simulink model "Test14Dof"  (R2024a)
settings: Solver=ode4  StartTime=0.0  StopTime=10.0  FixedStep=0.001  RelTol=1e-3
values from neighbouring files (symbols this model uses):
  EnvGrvty = 9.81    [Par.m]
  PlntBattChrgMax = 4.493    [Par.m]
  PlntBattNumCellSer = 96    [Par.m]
  PlntBattOpenCirctVolt = [3.17242 3.17242 3.17242 3.17242 3.17242 3.17242 3.17242;3.18272 3.18272 3.18272 3.18272 3.18272 3.18272 3.18272;3.19302 3.19302 3.19302 3.19302 3.19302 3.19302 3.19302;3.20331 3.20331 3.20331 3.20331 3.20331 3.20331 3.20331;3.21361 3.21361 3.21361 3.21361 3.21361 3.21361 3.21361;3.22391 3.22391 3.22391 3.22391 3.22391 3.22391 3.22391;3.23421 3.23421 3.23421 3.23421 3.23421 3.23421 3.23421;3.24451 ...(+5187 chars)    [Par.m]
  PlntBattSocInit = 0.6    [Par.m]
  PlntBattTempBpt = [-40 -30 -20 0 23 45 60]    [Par.m]
  PlntBattTempInitDegC = 25    [Par.m]
  PlntBattVoltSocBpt = [0 0.01 0.02 0.03 0.04 0.05 0.06 0.07 0.08 0.09 0.1 0.11 0.12 0.13 0.14 0.15 0.16 0.17 0.18 0.19 0.2 0.21 0.22 0.23 0.24 0.25 0.26 0.27 0.28 0.29 0.3 0.31 0.32 0.33 0.34 0.35 0.36 0.37 0.38 0.39 0.4 0.41 0.42 0.43 0.44 0.45 0.46 0.47 0.48 0.49 0.5 0.51 0.52 0.53 0.54 0.55 0.56 0.57 0.58 0.59 0.6 0.61 0.62 0.63 0.64 0.65 0.66 0.67 0.68 0.69 0.7 0.71 0.72 0.73 0.74 0.75 0.76 0.77 0.78 0.79 0.8 0.81  ...(+91 chars)    [Par.m]
  PlntDCDCVoltInit = 650    [Par.m]
  PlntDriveshftDamp = 100    [Par.m]
  PlntDriveshftStiff = 500    [Par.m]
  PlntEM1RotDamp = 0.001    [Par.m]
  PlntEM1RotInertia = 0.01    [Par.m]
  PlntEM2RotDamp = 0.001    [Par.m]
  PlntEM2RotInertia = 0.01    [Par.m]
  PlntEM3RotDamp = 0.001    [Par.m]
  PlntEM3RotInertia = 0.01    [Par.m]
  PlntEM4RotDamp = 0.001    [Par.m]
  PlntEM4RotInertia = 0.01    [Par.m]
  PlntEMWhlGearRatioFL = 11.04    [Par.m]
  PlntEMWhlGearRatioFR = 11.04    [Par.m]
  PlntEMWhlGearRatioRL = 11.04    [Par.m]
  PlntEMWhlGearRatioRR = 11.04    [Par.m]
  PlntSteerGearRatio = 52.025    [Par.m]
  PlntVehCGHgtAxl = 0.375    [Par.m]
  PlntVehDstCGFrntAxl = 1.61    [Par.m]
  PlntVehDstCGRearAxl = 1.39    [Par.m]
  PlntVehFrntUnsprgMass = 100    [Par.m]
  PlntVehInitLatPos = 0    [Par.m]
  PlntVehInitLatVel = 0    [Par.m]
  PlntVehInitLongPos = 0    [Par.m]
  PlntVehInitLongVel = 0    [Par.m]
  PlntVehInitPitchAng = 0    [Par.m]
  PlntVehInitPitchRate = 0    [Par.m]
  PlntVehInitRollAng = 0    [Par.m]
  PlntVehInitRollRate = 0    [Par.m]
  PlntVehInitVertPos = 0    [Par.m]
  PlntVehInitVertVel = 0    [Par.m]
  PlntVehInitYawAng = 0    [Par.m]
  PlntVehInitYawRate = 0    [Par.m]
  PlntVehMass = 2497    [Par.m]
  PlntVehPitchMomentInertia = 1922.7    [Par.m]
  PlntVehRearUnsprgMass = 100    [Par.m]
  PlntVehRollMomentInertia = 432.33333333333331    (= 432.333333333)    [Par.m]
  PlntVehTrckWdth = [1.685,1.685]    [Par.m]
  PlntVehYawMomentInertia = 2066    [Par.m]
  PlntWhlNumFrnt = 2    [Par.m]
  PlntWhlNumRear = 2    [Par.m]
  PlntWhlPrsFrnt = 220000    [Par.m]
  PlntWhlPrsRear = 220000    [Par.m]
undefined symbols (not defined in the file or in its folder): BdyFrm, InertFrm, PlntTrnsfrCaseAxlSpdLock, PlntTrnsfrCaseTrqSplitRatio
libraries: autolibsharedcoupling x12, autolibsharedcommon x12, autolibutils x10, autolibmappedmotor x4, autolibcoupling x4, matrix_library x4, vehdynlibsuspension x2, vehdynlibtire x2, vehdynlibtirecommon x2, vehdynlibsteering x2, shared6dof x2, autolibdatasheetbattery x1
(part 1 of 7)
settings Model: DataDictionary=VirtualVehicleTemplate.sldd  Creator=admin  LastModifiedBy=admin

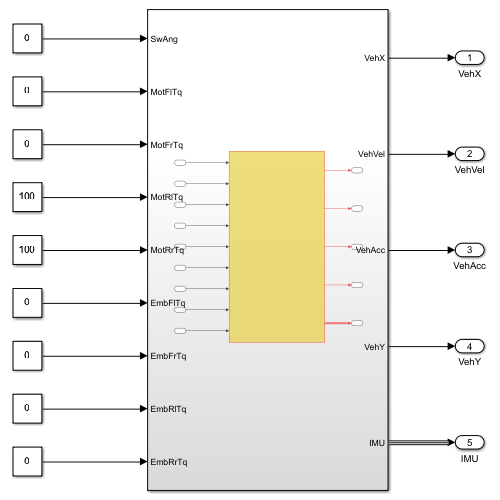
[thumbnail: Simulink's stored preview of the top-level diagram]
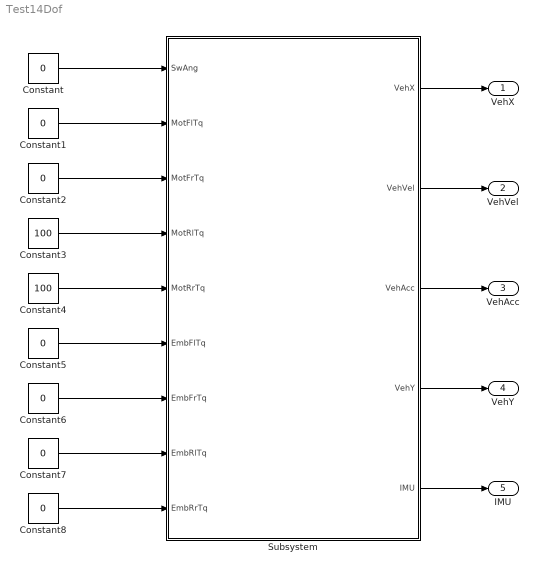
== system Test14Dof ==
  Constant{,1..2,5..8} (7 alike) : Constant  Value=0
  Constant3 : Constant  Value=100
  Constant4 : Constant  Value=100
  Subsystem : Subsystem
  VehX : Outport
  VehVel : Outport  Port=2
  VehAcc : Outport  Port=3
  VehY : Outport  Port=4
  IMU : Outport  Port=5
  wires:
  Subsystem/1(VehX) -> VehX/1
  Constant6/1 -> Subsystem/7(EmbFrTq)
  Constant5/1 -> Subsystem/6(EmbFlTq)
  Constant4/1 -> Subsystem/5(MotRrTq)
  Subsystem/3(VehAcc) -> VehAcc/1
  Constant2/1 -> Subsystem/3(MotFrTq)
  Constant/1 -> Subsystem/1(SwAng)
  Constant3/1 -> Subsystem/4(MotRlTq)
  Constant1/1 -> Subsystem/2(MotFlTq)
  Constant7/1 -> Subsystem/8(EmbRlTq)
  Subsystem/5(IMU) -> IMU/1
  Constant8/1 -> Subsystem/9(EmbRrTq)
  Subsystem/2(VehVel) -> VehVel/1
  Subsystem/4(VehY) -> VehY/1

== system Test14Dof/Subsystem ==
  SwAng : Inport
  MotFlTq : Inport  Port=2
  MotFrTq : Inport  Port=3
  MotRlTq : Inport  Port=4
  MotRrTq : Inport  Port=5
  EmbFlTq : Inport  Port=6
  EmbFrTq : Inport  Port=7
  EmbRlTq : Inport  Port=8
  EmbRrTq : Inport  Port=9
  Vehicle 14 DoF model : Subsystem
  VehX : Outport
  VehVel : Outport  Port=2
  VehAcc : Outport  Port=3
  VehY : Outport  Port=4
  IMU : Outport  Port=5
  wires:
  MotRrTq/1 -> Vehicle 14 DoF model/5(MotRrTq)
  MotFrTq/1 -> Vehicle 14 DoF model/3(MotFrTq)
  SwAng/1 -> Vehicle 14 DoF model/1(SwAng)
  MotRlTq/1 -> Vehicle 14 DoF model/4(MotRlTq)
  MotFlTq/1 -> Vehicle 14 DoF model/2(MotFlTq)
  EmbRlTq/1 -> Vehicle 14 DoF model/8(EmbRlTq)
  Vehicle 14 DoF model/3(VehAcc) -> VehAcc/1
  EmbFlTq/1 -> Vehicle 14 DoF model/6(EmbFlTq)
  Vehicle 14 DoF model/5(IMU) -> IMU/1
  EmbFrTq/1 -> Vehicle 14 DoF model/7(EmbFrTq)
  EmbRrTq/1 -> Vehicle 14 DoF model/9(EmbRrTq)
  Vehicle 14 DoF model/1(VehX) -> VehX/1
  Vehicle 14 DoF model/2(VehVel) -> VehVel/1
  Vehicle 14 DoF model/4(VehY) -> VehY/1

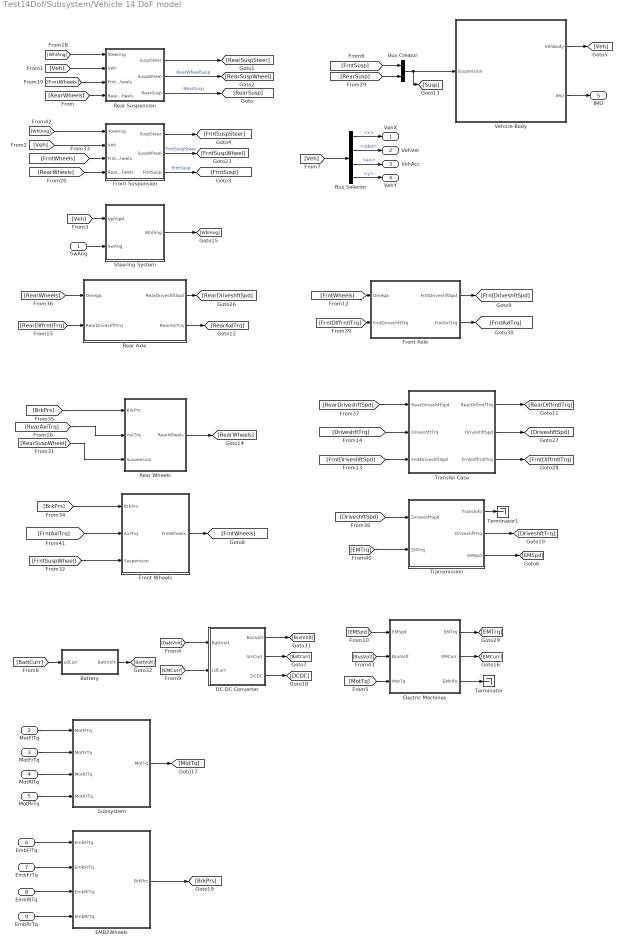
== system Test14Dof/Subsystem/Vehicle 14 DoF model ==
  SwAng : Inport
  MotFlTq : Inport  Port=2
  MotFrTq : Inport  Port=3
  MotRlTq : Inport  Port=4
  MotRrTq : Inport  Port=5
  EmbFlTq : Inport  Port=6
  EmbFrTq : Inport  Port=7
  EmbRlTq : Inport  Port=8
  EmbRrTq : Inport  Port=9
  Battery : Subsystem
  Bus Creator : BusCreator  Inputs=2
  Bus Selector : BusSelector  OutputSignals=BdyFrm.Cg.Disp.x,BdyFrm.Cg.Vel.xdot,BdyFrm.Cg.Acc.ax,BdyFrm.Cg.Disp.y
  DC-DC Converter : Subsystem
  EMB2Wheels : Subsystem
  Electric Machines : Subsystem
  Front Axle : Subsystem
  Front Suspension : Subsystem
  Front Wheels : Subsystem
  Rear Axle : Subsystem
  Rear Suspension : Subsystem
  Rear Wheels : Subsystem
  Steering System : Subsystem
  Subsystem : Subsystem
  Terminator : Terminator
  Terminator1 : Terminator
  Transfer Case : Subsystem
  Transmission : Subsystem
  Vehicle Body : Subsystem
  VehX : Outport
  VehVel : Outport  Port=2
  VehAcc : Outport  Port=3
  VehY : Outport  Port=4
  IMU : Outport  Port=5
  wires:
  EmbRrTq/1 -> EMB2Wheels/4(EmbRrTq)
  [FrntSuspWheel] -> Front Wheels/3(Suspension)
  Subsystem/1(MotTq) -> [MotTq]
  [FrntDiffrntlTrq] -> Front Axle/2(FrntDriveshftTrq)
  Transmission/3(EMSpd) -> [EMSpd]
  [FrntWheels] -> Rear Suspension/3(FrntWheels)
  MotRlTq/1 -> Subsystem/3(MotRlTq)
  EmbFlTq/1 -> EMB2Wheels/1(EmbFlTq)
  SwAng/1 -> Steering System/2(SwAng)
  [BrkPrs] -> Front Wheels/1(BrkPrs)
  [RearSusp] -> Bus Creator/2
  MotFrTq/1 -> Subsystem/2(MotFrTq)
  Electric Machines/1(EMTrq) -> [EMTrq]
  [RearDiffrntlTrq] -> Rear Axle/2(RearDriveshftTrq)
  Front Wheels/1(FrntWheels) -> [FrntWheels]
  Front Suspension/3(FrntSusp) -> [FrntSusp]  "FrntSusp"
  DC-DC Converter/2(SrcCurr) -> [BattCurr]
  [EMTrq] -> Transmission/2(EMTrq)
  [FrntWheels] -> Front Axle/1(Omega)
  [BusVolt] -> Electric Machines/2(BusVolt)
  [WhlAng] -> Rear Suspension/1(Steering)
  Front Suspension/2(SuspWheel) -> [FrntSuspWheel]  "FrntSuspSteer"
  Front Axle/1(FrntDriveshftSpd) -> [FrntDriveshftSpd]
  [BattCurr] -> Battery/1(LdCurr)
  Front Suspension/1(SuspSteer) -> [FrntSuspSteer]
  Vehicle Body/1(VehBody) -> [Veh]
  [MotTq] -> Electric Machines/3(MotTq)
  [RearWheels] -> Rear Axle/1(Omega)
  [FrntDriveshftSpd] -> Transfer Case/3(FrntDriveshftSpd)
  Battery/1(BattVolt) -> [BattVolt]
  Rear Axle/2(RearAxlTrq) -> [RearAxlTrq]
  [EMSpd] -> Electric Machines/1(EMSpd)
  [DriveshftSpd] -> Transmission/1(DriveshftSpd)
  [Veh] -> Steering System/1(VehSpd)
  [EMCurr] -> DC-DC Converter/2(LdCurr)
  Rear Wheels/1(RearWheels) -> [RearWheels]
  [RearWheels] -> Rear Suspension/4(RearWheels)
  Bus Creator/1 -> Vehicle Body/1(Suspension), [Susp]
  Transmission/2(DriveshftTrq) -> [DriveshftTrq]
  EmbFrTq/1 -> EMB2Wheels/2(EmbFrTq)
  Rear Suspension/2(SuspWheel) -> [RearSuspWheel]  "RearWheelSusp"
  [BattVolt] -> DC-DC Converter/1(BattVolt)
  [Veh] -> Rear Suspension/2(Veh)
  [DriveshftTrq] -> Transfer Case/2(DriveshftTrq)
  [BrkPrs] -> Rear Wheels/1(BrkPrs)
  MotRrTq/1 -> Subsystem/4(MotRrTq)
  Steering System/1(WhlAng) -> [WhlAng]
  Rear Suspension/1(SuspSteer) -> [RearSuspSteer]
  Transfer Case/2(DriveshftSpd) -> [DriveshftSpd]
  EMB2Wheels/1(BrkPrs) -> [BrkPrs]
  MotFlTq/1 -> Subsystem/1(MotFlTq)
  [RearDriveshftSpd] -> Transfer Case/1(RearDriveshftSpd)
  Transfer Case/3(FrntDiffrntlTrq) -> [FrntDiffrntlTrq]
  Electric Machines/2(EMCurr) -> [EMCurr]
  Front Axle/2(FrntAxlTrq) -> [FrntAxlTrq]
  [FrntSusp] -> Bus Creator/1
  EmbRlTq/1 -> EMB2Wheels/3(EmbRlTq)
  Rear Suspension/3(RearSusp) -> [RearSusp]  "RearSusp"
  DC-DC Converter/1(BusVolt) -> [BusVolt]
  [RearAxlTrq] -> Rear Wheels/2(AxlTrq)
  DC-DC Converter/3(DCDC) -> [DCDC]
  [RearSuspWheel] -> Rear Wheels/3(Suspension)
  Rear Axle/1(RearDriveshftSpd) -> [RearDriveshftSpd]
  [FrntAxlTrq] -> Front Wheels/2(AxlTrq)
  Transfer Case/1(RearDiffrntlTrq) -> [RearDiffrntlTrq]
  Transmission/1(TransInfo) -> Terminator1/1
  Electric Machines/3(EMInfo) -> Terminator/1
  [Veh] -> Front Suspension/2(Veh)
  [RearWheels] -> Front Suspension/4(RearWheels)
  [FrntWheels] -> Front Suspension/3(FrntWheels)
  [WhlAng] -> Front Suspension/1(Steering)
  [Veh] -> Bus Selector/1
  Bus Selector/1 -> VehX/1  "<x>"
  Bus Selector/2 -> VehVel/1  "<xdot>"
  Bus Selector/3 -> VehAcc/1  "<ax>"
  Bus Selector/4 -> VehY/1  "<y>"
  Vehicle Body/2(IMU) -> IMU/1

== system Test14Dof/Subsystem/Vehicle 14 DoF model/Battery ==
  LdCurr : Inport
  Constant : Constant  Value=27
  Fcn : Fcn  Expr=u+273
  Lithium Ion Battery Pack : autolibdatasheetbattery/Datasheet Battery  CapacityCtrl=Parameter  OutputVlt=Filtered  BattChargeMax=PlntBattChrgMax  Em=interp2(PlntBattTempBpt,PlntBattVoltSocBpt',PlntBattOpenCirctVolt,PlntBattTempInitDegC,PlntBattVoltSocBpt')'  CapLUTBp=PlntBattVoltSocBpt  RInt=PlntBattIntrnRes'  BattTempBp=PlntBattTempBpt+273.15  CapSOCBp=PlntBattSocBpt  Ns=PlntBattNumCellSer  Np=PlntBattNumCellPar  BattCapInit=PlntBattSocInit*PlntBattChrgMax  Tc=PlntBattTimeCnst  Vinit=interp2(PlntBattTempBpt,PlntBattVoltSocBpt,PlntBattOpenCirctVolt*PlntBattNumCellSer,PlntBattTempInitDegC,PlntBattSocInit)  RefBlkName='autolibdatasheetbattery/Datasheet Battery'
  BattVolt : Outport  VectorParamsAs1DForOutWhenUnconnected=off
  wires:
  Lithium Ion Battery Pack/2 -> BattVolt/1
  Constant/1 -> Fcn/1
  Fcn/1 -> Lithium Ion Battery Pack/2
  LdCurr/1 -> Lithium Ion Battery Pack/1  "TotalCurr"

== system Test14Dof/Subsystem/Vehicle 14 DoF model/DC-DC Converter ==
  BattVolt : Inport
  LdCurr : Inport  Port=2
  Bus Selector1 : BusSelector  OutputSignals=PwrLoss  OutputAsBus=on
  Constant3 : Constant  Value=PlntDCDCVoltInit  SampleTime=-1
  Cont LPF : autolibutils/Cont LPF  wc=1  AbsoluteTolerance=auto  aMode=6
  DC-DC Converter : autolibdcdc/Bidirectional DC-DC  Tc=PlntDCDCTimeCnst  Vinit=PlntDCDCVoltInit  Plimit=PlntDCDCPwrLmt  param_loss=Single efficiency measurement  eff=PlntDCDCEff  v_loss_bp=PlntDCDCLossV  i_loss_bp=PlntDCDCLossI  losses_table=PlntDCDCLossTbl  v_eff_bp=[200 400 600 800 1000]  i_eff_bp=[25 50 75 100]  efficiency_table=[96.2 98.1 98.7 99;98.1 99 99.4 99.5;98.7 99.4 99.6 99.7;99 99.5 99.7 99.8;99.2 99.6 99.7 99.8]  x_v_bp=[-1000 -800 -600 -400 -200 200 400 600 800 1000]  x_i_bp=[-100 -75 -50 -25 25 50 75 100]  x_losses_mat=[200.400801603196 225.67703109328 200.803212851408 201.612903225806 199.999999999997 200 225 200;160.320641282556 180.541624874624 201.005025125625 202.020202020203 200 200 180 160;180.541624874624 180.722891566267 181.086519114686 197.568389057748 194.999999999999 179.999999999997 180 180;201.005025125625 181.086519114686 202.020202020203 193.67991845056 190 200 179.999999999997 200;202.020202020203 197.568389057748 193.67991845056 197.505197505197 190 190 194.999999999999 200;200 194.999999999999 190 190 197.505197505197 193.67991845056 197.568389057748 202.020202020203;200 179.999999999997 200 190 193.67991845056 202.020202020203 181.086519114686 201.005025125625;180 180 179.999999999997 194.999999999999 197.568389057748 181.086519114686 180.722891566267 180.541624874624;160 180 200 200 202.020202020203 201.005025125625 180.541624874624 160.320641282556;200 225 200 199.999999999997 201.612903225806 200.803212851408 225.67703109328 200.400801603196]  RefBlkName='autolibdcdc/Bidirectional DC-DC'  CalLossMapData={'BaseCageProjectFileName','';'BaseMbcProjectFileName','';'TaskName','Calibrate Inverter Loss Map';'ChildTasks',{{'DataName','';'TaskName','Import Loss Data'},{'TaskName','Generate Response Models'},{'TaskName','Generate Calibration'},{'TaskName','Update Block Parameters'}}}
  BusVolt : Outport  VectorParamsAs1DForOutWhenUnconnected=off
  SrcCurr : Outport  Port=2  VectorParamsAs1DForOutWhenUnconnected=off
  Bus Element Out : Outport  Port=3  PortName=DCDC  Element=PwrELoss
  wires:
  Cont LPF/1 -> Bus Element Out/1
  Bus Selector1/1 -> Cont LPF/1
  LdCurr/1 -> DC-DC Converter/3
  BattVolt/1 -> DC-DC Converter/2
  DC-DC Converter/2 -> BusVolt/1
  DC-DC Converter/1 -> Bus Selector1/1
  Constant3/1 -> DC-DC Converter/1
  DC-DC Converter/3 -> SrcCurr/1

== system Test14Dof/Subsystem/Vehicle 14 DoF model/EMB2Wheels ==
  EmbFlTq : Inport
  EmbFrTq : Inport  Port=2
  EmbRlTq : Inport  Port=3
  EmbRrTq : Inport  Port=4
  Bus Creator : BusCreator  Inputs=4
  Gain{,1..3} (4 alike) : Gain
  Transfer Fcn{,1..3} (4 alike) : TransferFcn  Denominator=[0.01 1]
  BrkPrs : Outport
  wires:
  EmbRrTq/1 -> Gain1/1
  EmbFlTq/1 -> Gain/1
  EmbRlTq/1 -> Gain3/1
  EmbFrTq/1 -> Gain2/1
  Gain2/1 -> Transfer Fcn2/1
  Gain/1 -> Transfer Fcn/1
  Transfer Fcn3/1 -> Bus Creator/3
  Gain1/1 -> Transfer Fcn1/1
  Gain3/1 -> Transfer Fcn3/1
  Transfer Fcn/1 -> Bus Creator/1
  Transfer Fcn2/1 -> Bus Creator/2
  Transfer Fcn1/1 -> Bus Creator/4
  Bus Creator/1 -> BrkPrs/1

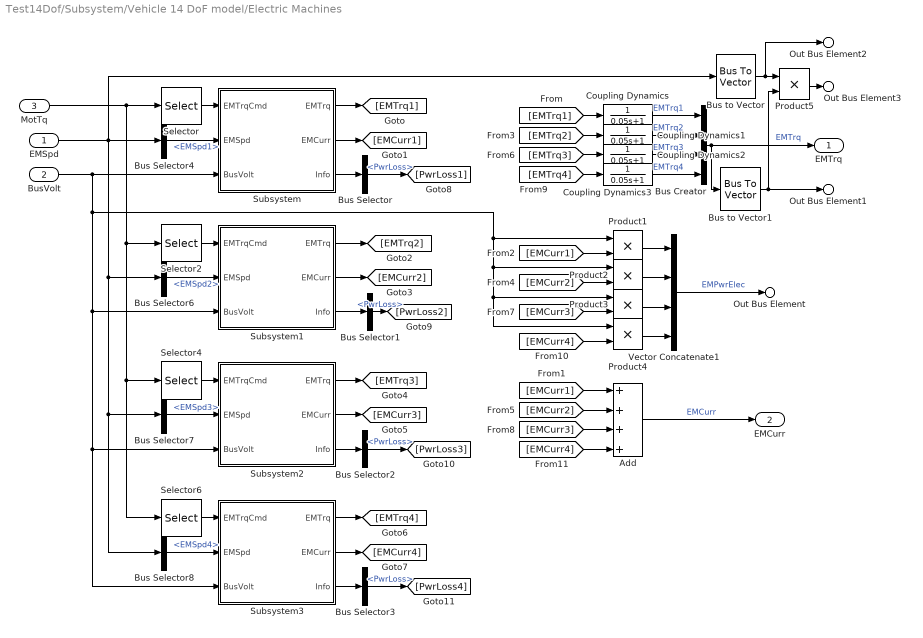
== system Test14Dof/Subsystem/Vehicle 14 DoF model/Electric Machines ==
  EMSpd : Inport
  BusVolt : Inport  Port=2
  MotTq : Inport  Port=3
  Add : Sum  Inputs=++++
  Bus Creator : BusCreator  Inputs=4
  Bus Selector{,1..3} (4 alike) : BusSelector  OutputSignals=PwrLoss
  Bus Selector4 : BusSelector  OutputSignals=EMSpd1
  Bus Selector6 : BusSelector  OutputSignals=EMSpd2
  Bus Selector7 : BusSelector  OutputSignals=EMSpd3
  Bus Selector8 : BusSelector  OutputSignals=EMSpd4
  Bus to Vector : BusToVector
  Bus to Vector1 : BusToVector
  Coupling Dynamics{,1..3} (4 alike) : TransferFcn  Denominator=[0.05 1]
  Product{1..5} (5 alike) : Product
  Selector : Selector  InputPortWidth=4  IndexOptions=Index vector (dialog)  Indices=[1]  OutputSizes=1
  Selector2 : Selector  InputPortWidth=4  IndexOptions=Index vector (dialog)  Indices=[2]  OutputSizes=1
  Selector4 : Selector  InputPortWidth=4  IndexOptions=Index vector (dialog)  Indices=[3]  OutputSizes=1
  Selector6 : Selector  InputPortWidth=4  IndexOptions=Index vector (dialog)  Indices=[4]  OutputSizes=1
  Subsystem : Subsystem
  Subsystem1 : Subsystem
  Subsystem2 : Subsystem
  Subsystem3 : Subsystem
  Vector Concatenate1 : Concatenate  NumInputs=4
  EMTrq : Outport
  EMCurr : Outport  Port=2
  Out Bus Element : Outport  Port=3  PortName=EMInfo  Element=EMPwrElec
  Out Bus Element1 : Outport  Port=3  PortName=EMInfo  Element=EMTrq
  Out Bus Element2 : Outport  Port=3  PortName=EMInfo  Element=EMSpd
  Out Bus Element3 : Outport  Port=3  PortName=EMInfo  Element=EMMechPwr
  wires:
  Bus Selector4/1 -> Subsystem/2(EMSpd)  "<EMSpd1>"
  [EMCurr2] -> Add/2
  Bus Selector1/1 -> [PwrLoss2]  "<PwrLoss>"
  [EMCurr3] -> Add/3
  [EMCurr2] -> Product2/2
  Product4/1 -> Vector Concatenate1/4
  Subsystem1/3(Info) -> Bus Selector1/1
  Bus Selector3/1 -> [PwrLoss4]  "<PwrLoss>"
  [EMCurr3] -> Product3/2
  Bus Selector6/1 -> Subsystem1/2(EMSpd)  "<EMSpd2>"
  Subsystem3/1(EMTrq) -> [EMTrq4]
  Subsystem2/3(Info) -> Bus Selector2/1
  Selector2/1 -> Subsystem1/1(EMTrqCmd)
  [EMTrq3] -> Coupling Dynamics2/1
  Selector4/1 -> Subsystem2/1(EMTrqCmd)
  Coupling Dynamics2/1 -> Bus Creator/3  "EMTrq3"
  Bus Selector/1 -> [PwrLoss1]  "<PwrLoss>"
  Subsystem3/3(Info) -> Bus Selector3/1
  Bus Selector2/1 -> [PwrLoss3]  "<PwrLoss>"
  Bus Selector7/1 -> Subsystem2/2(EMSpd)  "<EMSpd3>"
  Subsystem2/1(EMTrq) -> [EMTrq3]
  BusVolt/1 -> Subsystem/3(BusVolt), Subsystem1/3(BusVolt), Subsystem3/3(BusVolt), Subsystem2/3(BusVolt), Product1/1, Product4/1, Product3/1, Product2/1
  [EMCurr1] -> Product1/2
  Subsystem1/1(EMTrq) -> [EMTrq2]
  MotTq/1 -> Selector6/1, Selector4/1, Selector2/1, Selector/1
  Bus to Vector1/1 -> Product5/2, Out Bus Element1/1
  [EMCurr4] -> Add/4
  Product3/1 -> Vector Concatenate1/3
  [EMTrq4] -> Coupling Dynamics3/1
  Subsystem2/2(EMCurr) -> [EMCurr3]
  Subsystem/3(Info) -> Bus Selector/1
  Coupling Dynamics/1 -> Bus Creator/1  "EMTrq1"
  EMSpd/1 -> Bus Selector4/1, Bus Selector6/1, Bus Selector8/1, Bus Selector7/1, Bus to Vector/1
  Selector6/1 -> Subsystem3/1(EMTrqCmd)
  [EMCurr4] -> Product4/2
  Product5/1 -> Out Bus Element3/1
  Subsystem/1(EMTrq) -> [EMTrq1]
  Bus to Vector/1 -> Product5/1, Out Bus Element2/1
  Vector Concatenate1/1 -> Out Bus Element/1  "EMPwrElec"
  Product2/1 -> Vector Concatenate1/2
  Coupling Dynamics3/1 -> Bus Creator/4  "EMTrq4"
  Selector/1 -> Subsystem/1(EMTrqCmd)
  Subsystem/2(EMCurr) -> [EMCurr1]
  Product1/1 -> Vector Concatenate1/1
  Add/1 -> EMCurr/1  "EMCurr"
  [EMTrq1] -> Coupling Dynamics/1
  Bus Creator/1 -> Bus to Vector1/1, EMTrq/1  "EMTrq"
  [EMCurr1] -> Add/1
  Subsystem1/2(EMCurr) -> [EMCurr2]
  Bus Selector8/1 -> Subsystem3/2(EMSpd)  "<EMSpd4>"
  [EMTrq2] -> Coupling Dynamics1/1
  Subsystem3/2(EMCurr) -> [EMCurr4]
  Coupling Dynamics1/1 -> Bus Creator/2  "EMTrq2"

== system Test14Dof/Subsystem/Vehicle 14 DoF model/Front Axle ==
  Omega : Inport
  FrntDriveshftTrq : Inport  Port=2
  Bus Creator : BusCreator  Inputs=2
  Bus Selector : BusSelector  OutputSignals=Wheels.Omega
  Constant : Constant  Value=[0 0 0 0]
  Demux1 : Demux  Outputs=2
  Front Axle : Subsystem
  Front Axle Compliances : Subsystem
  Selector1 : Selector  InputPortWidth=4  IndexOptions=Index vector (dialog)  Indices=[3 4]  OutputSizes=1
  Subsystem : Subsystem
  FrntDriveshftSpd : Outport
  FrntAxlTrq : Outport  Port=2
  wires:
  Constant/1 -> Selector1/1
  Demux1/1 -> Front Axle/1(Prs1)
  Selector1/1 -> Demux1/1
  Demux1/2 -> Front Axle/2(Prs2)
  FrntDriveshftTrq/1 -> Front Axle/3(DriveshftTrq)
  Front Axle/2(DriveshftSpd) -> FrntDriveshftSpd/1
  Front Axle/3(Axl1Spd) -> Front Axle Compliances/1(RSpdL)
  Front Axle/4(Axl2Spd) -> Front Axle Compliances/2(RSpdR)
  Front Axle Compliances/2(RTrqR) -> Front Axle/5(Axl2Trq)
  Front Axle Compliances/1(RTrqL) -> Front Axle/4(Axl1Trq)
  Bus Selector/1 -> Subsystem/1(Omega)  "<Omega>"
  Omega/1 -> Bus Selector/1
  Subsystem/1(Omega_FL) -> Front Axle Compliances/3(OmegaL)
  Subsystem/2(Omega_FR) -> Front Axle Compliances/4(OmegaR)
  Front Axle Compliances/3(CTrqL) -> Bus Creator/1  "AxlTrqFL"
  Front Axle Compliances/4(CTrqR) -> Bus Creator/2  "AxlTrqFR"
  Bus Creator/1 -> FrntAxlTrq/1

== system Test14Dof/Subsystem/Vehicle 14 DoF model/Front Suspension ==
  Steering : Inport
  Veh : Inport  Port=2
  FrntWheels : Inport  Port=3
  RearWheels : Inport  Port=4
  Bus Creator : BusCreator  Inputs=2
  Bus Selector : BusSelector  OutputSignals=Wheels
  Bus Selector1 : BusSelector  OutputSignals=Wheels
  Kinematics and Compliance Independent Suspension : Subsystem
  Subsystem : Subsystem
  Susp2Wheel : Subsystem
  Wheel2Susp : Subsystem
  Wheel2SuspFrntOnly : Subsystem
  SuspSteer : Outport
  SuspWheel : Outport  Port=2
  FrntSusp : Outport  Port=3
  wires:
  Wheel2SuspFrntOnly/1(Wheels2Susp) -> SuspSteer/1
  FrntWheels/1 -> Bus Selector/1
  Kinematics and Compliance Independent Suspension/2(SuspensionFull) -> Susp2Wheel/1(Susp)
  Susp2Wheel/2(SuspFdbk) -> Wheel2Susp/3(SuspWheel)
  Bus Selector/1 -> Subsystem/1(Frnt), Susp2Wheel/3(Wheels), Wheel2SuspFrntOnly/2(Wheels)  "<Wheels>"
  Veh/1 -> Kinematics and Compliance Independent Suspension/2(Vehicle), Wheel2Susp/1(Veh), Wheel2SuspFrntOnly/1(Veh)
  Bus Creator/1 -> FrntSusp/1  "FrntSusp"
  RearWheels/1 -> Bus Selector1/1
  Subsystem/1(Wheels) -> Wheel2Susp/2(Wheels)
  Wheel2Susp/1(Wheels2Susp) -> Kinematics and Compliance Independent Suspension/3(Wheel), Susp2Wheel/2(WheelSusp)
  Steering/1 -> Kinematics and Compliance Independent Suspension/1(Steering)
  Bus Selector1/1 -> Subsystem/2(Rear)  "<Wheels>"
  Susp2Wheel/1(SuspWheel) -> SuspWheel/1, Bus Creator/2, Wheel2SuspFrntOnly/3(SuspWheel)  "FrntSuspWheel"
  Kinematics and Compliance Independent Suspension/1(Suspension) -> Bus Creator/1  "FrntSuspChassis"

== system Test14Dof/Subsystem/Vehicle 14 DoF model/Front Wheels ==
  BrkPrs : Inport
  AxlTrq : Inport  Port=2
  Suspension : Inport  Port=3
  Bus Creator1 : BusCreator  Inputs=2
  Bus Creator3 : BusCreator  Inputs=3
  Bus Selector : BusSelector  OutputSignals=Vx,Vy,WhlAng,YawRate,Fext
  Bus Creator : Subsystem
  Bus to Vector : BusToVector
  Constant : Constant  Value=[0.9 0.9 0.9 0.9]
  Constant1 : Constant  Value=[0 0 0 0]
  Constant2 : Constant  Value=repmat(eye(3),1,1,4)
  Front Friction : Subsystem
  Front Ground : Subsystem
  MF Tires Vector : Subsystem  VariantControl=MF Tires Vector
  Reshape : Reshape
  Selector : Selector  NumberOfDimensions=2  InputPortWidth=3  IndexOptions=Index vector (dialog),Select all  Indices=[1],1  OutputSizes=1,1
  Selector1 : Selector  NumberOfDimensions=3  IndexOptions=Index vector (dialog),Index vector (dialog),Index vector (dialog)  Indices=[1 2 3],[1 2 3],[1 2]  OutputSizes=1,1,1
  Selector4 : Selector  InputPortWidth=4  IndexOptions=Index vector (dialog)  Indices=[1 2]  OutputSizes=1
  Subsystem : Subsystem
  FrntWheels : Outport
  wires:
  Subsystem/2(ScaleFctrs) -> MF Tires Vector/9(ScaleFctrs)
  AxlTrq/1 -> Bus to Vector/1
  Bus to Vector/1 -> MF Tires Vector/2(AxlTrq)
  Selector1/1 -> Bus Creator3/3  "DCM"
  Bus Selector/2 -> MF Tires Vector/4(Vy)  "<Vy>"
  Front Friction/1(y) -> Subsystem/2(lamda_mu_y), Subsystem/1(lamda_mu_x), Bus Creator3/1  "mu"
  Reshape/1 -> MF Tires Vector/5(Camber)
  Subsystem/1(Prs) -> MF Tires Vector/8(Prs)
  Front Ground/1(y) -> MF Tires Vector/10(Gnd), Bus Creator3/2  "z"
  Selector4/1 -> MF Tires Vector/1(BrkPrs)
  Bus Selector/5 -> MF Tires Vector/7(Fext)  "<Fext>"
  Bus Selector/1 -> MF Tires Vector/3(Vx)  "<Vx>"
  Bus Selector/3 -> Selector/1  "<WhlAng>"
  Suspension/1 -> Bus Selector/1
  BrkPrs/1 -> Selector4/1
  Bus Selector/4 -> MF Tires Vector/6(YawRate)  "<YawRate>"
  Selector/1 -> Reshape/1
  Constant1/1 -> Front Ground/1(u)
  Constant/1 -> Front Friction/1(u)
  Constant2/1 -> Selector1/1
  Bus Creator1/1 -> FrntWheels/1
  Bus Creator/1(Wheels) -> Bus Creator1/1  "Wheels"
  MF Tires Vector/1(Wheels) -> Bus Creator/1(Info)
  Bus Creator3/1 -> Bus Creator1/2  "Gnd"

== system Test14Dof/Subsystem/Vehicle 14 DoF model/Rear Axle ==
  Omega : Inport
  RearDriveshftTrq : Inport  Port=2
  Bus Creator : BusCreator  Inputs=2
  Bus Selector : BusSelector  OutputSignals=Wheels.Omega
  Constant : Constant  Value=[0 0 0 0]
  Demux1 : Demux  Outputs=2
  Rear Axle : Subsystem
  Selector1 : Selector  InputPortWidth=4  IndexOptions=Index vector (dialog)  Indices=[3 4]  OutputSizes=1
  Subsystem : Subsystem
  Subsystem1 : Subsystem
  Terminator1 : Terminator
  RearDriveshftSpd : Outport
  RearAxlTrq : Outport  Port=2
  wires:
  Subsystem/1(RTrqL) -> Rear Axle/4(Axl1Trq)
  Bus Selector/1 -> Subsystem1/1(Omega)  "<Omega>"
  Omega/1 -> Bus Selector/1
  Demux1/2 -> Rear Axle/2(Prs2)
  Subsystem/2(RTrqR) -> Rear Axle/5(Axl2Trq)
  Selector1/1 -> Demux1/1
  RearDriveshftTrq/1 -> Rear Axle/3(DriveshftTrq)
  Demux1/1 -> Rear Axle/1(Prs1)
  Rear Axle/3(Axl1Spd) -> Subsystem/1(RSpdL)
  Rear Axle/4(Axl2Spd) -> Subsystem/2(RSpdR)
  Subsystem1/1(Omega_RL) -> Subsystem/3(OmegaL)
  Subsystem1/2(Omega_RR) -> Subsystem/4(OmegaR)
  Rear Axle/2(DriveshftSpd) -> RearDriveshftSpd/1
  Bus Creator/1 -> RearAxlTrq/1
  Subsystem/3(CTrqL) -> Bus Creator/1  "AxlTrqRL"
  Subsystem/4(CTrqR) -> Bus Creator/2  "AxlTrqRR"
  Constant/1 -> Selector1/1
  Rear Axle/1(Info) -> Terminator1/1

== system Test14Dof/Subsystem/Vehicle 14 DoF model/Rear Suspension ==
  note: Copyright 2022-2023 The MathWorks, Inc.
  Steering : Inport
  Veh : Inport  Port=2
  FrntWheels : Inport  Port=3
  RearWheels : Inport  Port=4
  Bus Creator : BusCreator  Inputs=2
  Bus Selector : BusSelector  OutputSignals=Wheels
  Bus Selector1 : BusSelector  OutputSignals=Wheels
  Kinematics and Compliance Independent Suspension : Subsystem
  Subsystem : Subsystem
  Susp2Wheel : Subsystem
  Wheel2Susp : Subsystem
  Wheel2SuspRearOnly : Subsystem
  SuspSteer : Outport
  SuspWheel : Outport  Port=2
  RearSusp : Outport  Port=3
  wires:
  Bus Selector1/1 -> Subsystem/2(Rear), Susp2Wheel/3(Wheels), Wheel2SuspRearOnly/2(Wheels)  "<Wheels>"
  Subsystem/1(Wheels) -> Wheel2Susp/2(Wheels)
  Kinematics and Compliance Independent Suspension/2(SuspensionFull) -> Susp2Wheel/1(Susp)
  RearWheels/1 -> Bus Selector1/1
  Susp2Wheel/2(SuspFdbk) -> Wheel2Susp/3(SuspWheel)
  Bus Creator/1 -> RearSusp/1  "RearSusp"
  Steering/1 -> Kinematics and Compliance Independent Suspension/1(Steering)
  Susp2Wheel/1(SuspWheel) -> Wheel2SuspRearOnly/3(SuspWheel), SuspWheel/1, Bus Creator/2  "RearSuspWheel"
  Wheel2SuspRearOnly/1(Wheels2Susp) -> SuspSteer/1
  Wheel2Susp/1(Wheels2Susp) -> Kinematics and Compliance Independent Suspension/3(Wheel), Susp2Wheel/2(WheelSusp)
  Bus Selector/1 -> Subsystem/1(Frnt)  "<Wheels>"
  FrntWheels/1 -> Bus Selector/1
  Kinematics and Compliance Independent Suspension/1(Suspension) -> Bus Creator/1  "RearSuspChassis"
  Veh/1 -> Kinematics and Compliance Independent Suspension/2(Vehicle), Wheel2Susp/1(Veh), Wheel2SuspRearOnly/1(Veh)

== system Test14Dof/Subsystem/Vehicle 14 DoF model/Rear Wheels ==
  BrkPrs : Inport
  AxlTrq : Inport  Port=2
  Suspension : Inport  Port=3
  Bus Creator1 : BusCreator  Inputs=2
  Bus Creator3 : BusCreator  Inputs=3
  Bus Selector : BusSelector  OutputSignals=Vx,Vy,WhlAng,YawRate,Fext
  Bus Creator : Subsystem
  Bus to Vector : BusToVector
  Constant : Constant  Value=[0.9 0.9 0.9 0.9]
  Constant1 : Constant  Value=[0 0 0 0]
  Constant2 : Constant  Value=repmat(eye(3),1,1,4)
  MF Tires Vector : Subsystem  VariantControl=MF Tires Vector
  Rear Friction : Subsystem
  Rear Ground : Subsystem
  Reshape : Reshape
  Selector : Selector  NumberOfDimensions=2  InputPortWidth=3  IndexOptions=Index vector (dialog),Select all  Indices=[1],1  OutputSizes=1,1
  Selector1 : Selector  NumberOfDimensions=3  IndexOptions=Index vector (dialog),Index vector (dialog),Index vector (dialog)  Indices=[1 2 3],[1 2 3],[3 4]  OutputSizes=1,1,1
  Selector4 : Selector  InputPortWidth=4  IndexOptions=Index vector (dialog)  Indices=[3 4]  OutputSizes=1
  Subsystem : Subsystem
  RearWheels : Outport  VectorParamsAs1DForOutWhenUnconnected=off
  wires:
  BrkPrs/1 -> Selector4/1
  Rear Friction/1(y) -> Subsystem/2(lamda_mu_y), Subsystem/1(lamda_mu_x), Bus Creator3/1  "mu"
  AxlTrq/1 -> Bus to Vector/1
  Rear Ground/1(y) -> MF Tires Vector/10(Gnd), Bus Creator3/2  "z"
  Selector1/1 -> Bus Creator3/3  "DCM"
  Selector/1 -> Reshape/1
  Bus Selector/4 -> MF Tires Vector/6(YawRate)  "<YawRate>"
  Bus Selector/5 -> MF Tires Vector/7(Fext)  "<Fext>"
  Bus Selector/2 -> MF Tires Vector/4(Vy)  "<Vy>"
  Suspension/1 -> Bus Selector/1
  Bus Selector/3 -> Selector/1  "<WhlAng>"
  Bus Selector/1 -> MF Tires Vector/3(Vx)  "<Vx>"
  Bus to Vector/1 -> MF Tires Vector/2(AxlTrq)
  Selector4/1 -> MF Tires Vector/1(BrkPrs)
  Subsystem/1(Prs) -> MF Tires Vector/8(Prs)
  Subsystem/2(ScaleFctrs) -> MF Tires Vector/9(ScaleFctrs)
  MF Tires Vector/1(Wheels) -> Bus Creator/1(Info)
  Bus Creator/1(Wheels) -> Bus Creator1/1  "Wheels"
  Bus Creator3/1 -> Bus Creator1/2  "Gnd"
  Bus Creator1/1 -> RearWheels/1
  Constant1/1 -> Rear Ground/1(u)
  Constant/1 -> Rear Friction/1(u)
  Constant2/1 -> Selector1/1
  Reshape/1 -> MF Tires Vector/5(Camber)

== system Test14Dof/Subsystem/Vehicle 14 DoF model/Steering System ==
  VehSpd : Inport
  SwAng : Inport  Port=2
  Bus Creator1 : BusCreator  Inputs=2
  Bus Creator2 : BusCreator  Inputs=1
  Bus Creator3 : BusCreator  Inputs=2
  Bus Creator4 : BusCreator  Inputs=1
  Bus Creator5 : BusCreator  Inputs=2
  Bus Selector : BusSelector  OutputSignals=BdyFrm.Cg.Vel.xdot
  Bus Selector1 : BusSelector  OutputSignals=Front.WhlAng.FL,Front.WhlAng.FR,Rear.WhlAng.RL,Rear.WhlAng.RR  OutputAsBus=on
  Bus to Vector : BusToVector
  Constant : Constant  Value=0  SampleTime=-1
  Front Steering : vehdynlibsteering/Mapped Steering  SpdDpd=on  IndexType=Rack travel displacement  GrType=Constant  StrgAngBpts=[-1.5*pi 1.5*pi]  RackDispBpts=PlntSteerRackDispBpt  Gr=PlntSteerGearRatio  GrTbl=[9.87 9.87 7.16 7.16 9.87 9.87]*2*pi  WhlLftTbl=PlntSteerLftWhlAngTbl  WhlRghtTbl=PlntSteerRghtWhlAngTbl  VehSpdBpts=[-1 1]  SpdFctTbl=[1 1]  aMode=2
  Rear Steering : vehdynlibsteering/Mapped Steering  SpdDpd=on  IndexType=Rack travel displacement  GrType=Constant  StrgAngBpts=[-1.5*pi 1.5*pi]  RackDispBpts=PlntSteerRackDispBpt  Gr=PlntSteerGearRatio/10  GrTbl=[9.87 9.87 7.16 7.16 9.87 9.87]*2*pi  WhlLftTbl=PlntSteerLftWhlAngTbl  WhlRghtTbl=PlntSteerRghtWhlAngTbl  VehSpdBpts=[-1 1]  SpdFctTbl=[1 1]  aMode=2
  Terminator : Terminator
  Terminator1 : Terminator
  WhlAng : Outport  VectorParamsAs1DForOutWhenUnconnected=off
  wires:
  Rear Steering/1 -> Terminator1/1
  Bus Creator5/1 -> Bus Creator4/1  "WhlAng"
  Front Steering/3 -> Bus Creator3/2  "FR"
  Front Steering/1 -> Terminator/1
  Rear Steering/3 -> Bus Creator5/2  "RR"
  Front Steering/2 -> Bus Creator3/1  "FL"
  Bus Selector/1 -> Rear Steering/2, Front Steering/2  "<xdot>"
  Bus Selector1/1 -> Bus to Vector/1
  Bus Creator3/1 -> Bus Creator2/1  "WhlAng"
  Bus to Vector/1 -> WhlAng/1
  Bus Creator1/1 -> Bus Selector1/1
  Rear Steering/2 -> Bus Creator5/1  "RL"
  VehSpd/1 -> Bus Selector/1
  Bus Creator2/1 -> Bus Creator1/1  "Front"
  Constant/1 -> Rear Steering/1
  Bus Creator4/1 -> Bus Creator1/2  "Rear"
  SwAng/1 -> Front Steering/1

== system Test14Dof/Subsystem/Vehicle 14 DoF model/Subsystem ==
  MotFlTq : Inport
  MotFrTq : Inport  Port=2
  MotRlTq : Inport  Port=3
  MotRrTq : Inport  Port=4
  Bus Creator : BusCreator  Inputs=4
  MotTq : Outport
  wires:
  MotFlTq/1 -> Bus Creator/1
  MotRlTq/1 -> Bus Creator/3
  MotFrTq/1 -> Bus Creator/2
  Bus Creator/1 -> MotTq/1
  MotRrTq/1 -> Bus Creator/4

== system Test14Dof/Subsystem/Vehicle 14 DoF model/Transfer Case ==
  RearDriveshftSpd : Inport
  DriveshftTrq : Inport  Port=2
  FrntDriveshftSpd : Inport  Port=3
  Bus Creator : BusCreator  Inputs=2
  Constant : Constant  Value=PlntTrnsfrCaseTrqSplitRatio  SampleTime=-1
  Constant1 : Constant  Value=PlntTrnsfrCaseAxlSpdLock  SampleTime=-1
  DriveshftTrq Routing : Subsystem
  Subsystem : Subsystem
  RearDiffrntlTrq : Outport  VectorParamsAs1DForOutWhenUnconnected=off
  DriveshftSpd : Outport  Port=2  VectorParamsAs1DForOutWhenUnconnected=off
  FrntDiffrntlTrq : Outport  Port=3  VectorParamsAs1DForOutWhenUnconnected=off
  wires:
  Constant/1 -> Subsystem/1(TrqSplitRatio)
  Constant1/1 -> Subsystem/2(SpdLock)
  DriveshftTrq/1 -> DriveshftTrq Routing/2(DriveshftTrq)
  Subsystem/3(RearDiffrntlTrq) -> DriveshftTrq Routing/3("TrnsfrCaseRearTrq ")
  Subsystem/2(FrntDiffrntlTrq) -> DriveshftTrq Routing/1(TrnsfrCaseFrntTrq)
  FrntDriveshftSpd/1 -> Bus Creator/1, Subsystem/3(FrntDiffrntlSpd)  "FrntDriveshftSpd"
  DriveshftTrq Routing/2(TrnsfrCaseTrq) -> Subsystem/4(DriveshftTrq)
  DriveshftTrq Routing/3(RearDiffrntlTrq) -> RearDiffrntlTrq/1
  RearDriveshftSpd/1 -> Bus Creator/2, Subsystem/5(RearDiffrntlSpd)  "RearDriveshftSpd"
  Bus Creator/1 -> DriveshftSpd/1
  DriveshftTrq Routing/1(FrntDiffrntlTrq) -> FrntDiffrntlTrq/1

== system Test14Dof/Subsystem/Vehicle 14 DoF model/Transmission ==
  DriveshftSpd : Inport
  EMTrq : Inport  Port=2
  BEV4 : Subsystem
  TransInfo : Outport
  DriveshftTrq : Outport  Port=2
  EMSpd : Outport  Port=3
  wires:
  EMTrq/1 -> BEV4/1(EMTrq)
  DriveshftSpd/1 -> BEV4/2(DriveshftSpd)
  BEV4/1(EMSpd) -> EMSpd/1
  BEV4/2(DriveshftTrq) -> DriveshftTrq/1
  BEV4/3(TransInfo) -> TransInfo/1

== system Test14Dof/Subsystem/Vehicle 14 DoF model/Vehicle Body ==
  Suspension : Inport
  Subsystem : Subsystem
  Vehicle 6DOF : Subsystem
  Bus Element Out : Outport  PortName=VehBody
  IMU : Outport  Port=2
  wires:
  Suspension/1 -> Vehicle 6DOF/1(Suspension)
  Vehicle 6DOF/1(VehBody) -> Bus Element Out/1, Subsystem/1(Veh)
  Subsystem/1(IMU) -> IMU/1

== system Test14Dof/Subsystem/Vehicle 14 DoF model/Electric Machines/Subsystem ==
  EMTrqCmd : Inport
  EMSpd : Inport  Port=2
  BusVolt : Inport  Port=3
  Mapped Motor : autolibmappedmotor/Mapped Motor  port_config=Speed  param_by=Tabulated torque-speed envelope  w_t=PlntEM1Spd  T_t=PlntEM1Trq  torque_max=0.1  power_max=30  Tc=PlntEM1TimeCnst  param_loss=Tabulated efficiency data  eff=100  w_eff=375  T_eff=0.08  Piron=0  Pbase=0  w_eff_bp=PlntEM1SpdEff  T_eff_bp=PlntEM1TrqEff  Temp_eff_bp=Temp_eff_bp  losses_table=PlntEM1TrqLossTbl  losses_table_3d=losses_table_3d  efficiency_table=PlntEM1EffTbl  efficiency_table_3d=efficiency_table_3d  J=5e-6  b=1e-5  omega_o=0  T_t_extended=[125.931348721462 137.379653150686 151.117618465755 167.90846496195 188.897023082193 215.882312093935 251.862697442924 302.235236931509 377.794046164387 450 450 450 450 450 450 450 450 450 377.794046164387 302.235236931509 251.862697442924 215.882312093935 188.897023082193 167.90846496195 151.117618465755 137.379653150686 125.931348721462]  w_t_extended=[-1675.51608191456 -1535.88974175501 -1396.26340159546 -1256.63706143592 -1117.01072127637 -977.384381116825 -837.758040957278 -698.131700797732 -558.505360638185 -468.888888888889 -418.879020478639 -279.252680319093 -139.626340159546 0 139.626340159546 279.252680319093 418.879020478639 468.888888888889 558.505360638185 698.131700797732 837.758040957278 977.384381116825 1117.01072127637 1256.63706143592 1396.26340159546 1535.88974175501 1675.51608191456]  KLossIron=0  KLossCopper=0  x_w_eff_vec=[-1675.51608191456 -1535.88974175501 -1396.26340159546 -1256.63706143592 -1117.01072127637 -977.384381116825 -837.758040957278 -698.131700797732 -558.505360638185 -468.888888888889 -418.879020478639 -279.252680319093 -139.626340159546 0 139.626340159546 279.252680319093 418.879020478639 468.888888888889 558.505360638185 698.131700797732 837.758040957278 977.384381116825 1117.01072127637 1256.63706143592 1396.26340159546 1535.88974175501 1675.51608191456]  x_T_eff_vec=[-450 -405 -360 -315 -270 -225 -180 -135 -90 -45 0 45 90 135 180 225 270 315 360 405 450]  x_tmp_eff_vec=[233.15 293.15 373.15]  x_losses_mat=[56751.351161622 51076.2160454598 45401.0809292976 39725.9458131354 34050.8106969732 28375.675580811 22700.5404646488 17025.4053484866 14913.9343555032 12274.1294372811 0 10555.7513160617 13571.6802635079 15833.6269740925 21111.5026321234 26389.3782901542 31667.2539481851 36945.1296062159 42223.0052642468 47500.8809222776 52778.7565803085;52022.0718981535 46819.8647083382 41617.6575185228 36415.4503287075 31213.2431388921 26011.0359490768 20808.8287592614 15606.6215694461 12020.0066746044 11251.2853175076 0 9676.10537305656 11058.4061406361 14514.1580595848 19352.2107461131 24190.2634326414 29028.3161191697 33866.3688056979 38704.4214922262 43542.4741787545 48380.5268652828;47292.792634685 42563.5133712165 37834.234107748 33104.9548442795 28375.675580811 23646.3963173425 18917.117053874 14187.8377904055 10927.2787950949 10228.4411977342 0 8796.45943005142 10053.0964914873 13194.6891450771 17592.9188601028 21991.1485751285 26389.3782901542 30787.60800518 35185.8377202057 39584.0674352314 43982.2971502571;42563.5133712165 38307.1620340949 34050.8106969732 29794.4593598516 25538.1080227299 21281.7566856083 17025.4053484866 12769.054011365 11185.4507666274 9205.59707796079 0 7916.81348704628 10178.7601976309 11875.2202305694 15833.6269740925 19792.0337176157 23750.4404611388 27708.847204662 31667.2539481851 35625.6606917082 39584.0674352314;37834.234107748 34050.8106969732 30267.3872861984 26483.9638754236 22700.5404646488 18917.117053874 15133.6936430992 11350.2702323244 9942.62290366878 8182.75295818737 0 7037.16754404114 9047.7868423386 10555.7513160617 14074.3350880823 17592.9188601028 21111.5026321234 24630.086404144 28148.6701761645 31667.2539481851 35185.8377202057;33104.9548442795 29794.4593598516 26483.9638754236 23173.4683909957 19862.9729065677 16552.4774221398 15298.1903131329 11473.6427348497 9773.84381116825 8377.58040957278 0 7037.16754404114 8796.45943005142 10555.7513160617 14074.3350880823 15393.80400259 18472.564803108 21551.325603626 24630.086404144 27708.847204662 30787.60800518;28375.675580811 25538.1080227299 22700.5404646488 19862.9729065677 17025.4053484866 16390.9181926424 14913.9343555032 11185.4507666274 10281.575957203 8275.41479482189 0 6785.84013175395 9047.7868423386 10178.7601976309 13571.6802635079 15079.644737231 15833.6269740925 18472.564803108 21111.5026321234 23750.4404611388 26389.3782901542;31070.6965739649 27963.6269165685 21854.5575901899 19122.7378914161 16390.9181926424 15535.3482869825 12428.278629586 10471.975511966 8567.97996433581 6896.17899568491 0 5654.86677646163 7539.8223686155 9424.77796076938 11309.7335529233 14137.1669411541 15079.644737231 17592.9188601028 20106.1929829747 25446.9004940773 28274.3338823081;34271.9198573432 30844.7278716089 27417.5358858746 19547.6876223365 16755.1608191456 13962.6340159546 11170.1072127637 10281.575957203 8182.75295818737 6283.18530717959 0 5026.54824574367 7037.16754404114 9047.78684233861 10053.0964914873 12566.3706143592 15079.644737231 17592.9188601028 24127.4315795696 27143.3605270158 30159.289474462;34348.8372093023 30913.9534883721 27479.0697674419 20140.9090909091 17263.6363636364 14386.3636363636 11509.0909090909 8631.81818181819 6869.76744186047 5275 0 4220 5908 7596 10128 12660 15192 17724 23632 26586 29540;35903.9160410262 32313.5244369236 24548.2588745621 21479.7265152418 15422.3639358044 12851.9699465037 10281.575957203 9205.59707796079 6137.06471864053 4712.38898038469 0 3769.91118430775 5277.87565803085 7916.81348704628 9047.7868423386 11309.7335529233 13571.6802635079 18472.564803108 21111.5026321234 27143.3605270158 30159.289474462;27584.7159827396 24826.2443844657 19148.7552218806 16755.1608191456 12274.1294372811 10228.4411977342 8182.75295818737 6137.06471864053 4787.18880547016 3544.36094251156 0 2764.60153515902 4021.23859659494 5277.87565803085 7037.16754404114 8796.45943005142 10555.7513160617 14074.3350880823 16084.9543863797 20357.5203952619 22619.4671058465;26927.9370307696 19868.4508362165 15873.3102497169 ...(+4614 chars)]  x_losses_mat_3d=cat(3,[2 2 2 2 2 2 2 2 2 2 2 2 2 2 2 2 2 2 2 2 2;2 2 2 2 2 2 2 2 2 2 2 2 2 2 2 2 2 2 2 2 2;2 2 2 2 2 2 2 2 2 2 2 2 2 2 2 2 2 2 2 2 2;2 2 2 2 2 2 2 2 2 2 2 2 2 2 2 2 2 2 2 2 2;2 2 2 2 2 2 2 2 2 2 2 2 2 2 2 2 2 2 2 2 2;2 2 2 2 2 2 2 2 2 2 2 2 2 2 2 2 2 2 2 2 2;2 2 2 2 2 2 2 2 2 2 2 2 2 2 2 2 2 2 2 2 2;2 2 2 2 2 2 2 2 2 2 2 2 2 2 2 2 2 2 2 2 2;2 2 2 2 2 2 2 2 2 2 2 2 2 2 2 2 2 2 2 2 2;2 2 2 2 2 2 2 2 2 2 2 2 2 2 2 2 2 2 2 2 2;2 2 2 2 2 2 2 2 2 2 2 2 2 2 2 2 2 2 2 2 2;2 2 2 2 2 2 2 2 2 2 2 2 2 2 2 2 2 2 2 2 2;2 2 2 2 2 2 2 2 2 2 2 2 2 2 2 2 2 2 2 2 2;2 2 2 2 2 2 2 2 2 2 2 2 2 2 2 2 2 2 2 2 2;2 2 2 2 2 2 2 2 2 2 2 2 2 2 2 2 2 2 2 2 2;2 2 2 2 2 2 2 2 2 2 2 2 2 2 2 2 2 2 2 2 2;2 2 2 2 2 2 2 2 2 2 2 2 2 2 2 2 2 2 2 2 2;2 2 2 2 2 2 2 2 2 2 2 2 2 2 2 2 2 2 2 2 2;2 2 2 2 2 2 2 2 2 2 2 2 2 2 2 2 2 2 2 2 2;2 2 2 2 2 2 2 2 2 2 2 2 2 2 2 2 2 2 2 2 2;2 2 2 2 2 2 2 2 2 2 2 2 2 2 2 2 2 2 2 2 2;2 2 2 2 2 2 2 2 2 2 2 2 2 2 2 2 2 2 2 2 2;2 2 2 2 2 2 2 2 2 2 2 2 2 2 2 2 2 2 2 2 2;2 2 2 2 2 2 2 2 2 2 2 2 2 2 2 2 2 2 2 2 2;2 2 2 2 2 2 2 2 2 2 2 2 2 2 2 2 2 2 2 2 2;2 2 2 2 2 2 2 2 2 2 2 2 2 2 2 2 2 2 2 2 2;2 2 2 2 2 2 2 2 2 2 2 2 2 2 2 2 2 2 2 2 2],[1.5 1.5 1.5 1.5 1.5 1.5 1.5 1.5 1.5 1.5 1.5 1.5 1.5 1.5 1.5 1.5 1.5 1.5 1.5 1.5 1.5;1.5 1.5 1.5 1.5 1.5 1.5 1.5 1.5 1.5 1.5 1.5 1.5 1.5 1.5 1.5 1.5 1.5 1.5 1.5 1.5 1.5;1.5 1.5 1.5 1.5 1.5 1.5 1.5 1.5 1.5 1.5 1.5 1.5 1.5 1.5 1.5 1.5 1.5 1.5 1.5 1.5 1.5;1.5 1.5 1.5 1.5 1.5 1.5 1.5 1.5 1.5 1.5 1.5 1.5 1.5 1.5 1.5 1.5 1.5 1.5 1.5 1.5 1.5;1.5 1.5 1.5 1.5 1.5 1.5 1.5 1.5 1.5 1.5 1.5 1.5 1.5 1.5 1.5 1.5 1.5 1.5 1.5 1.5 1.5;1.5 1.5 1.5 1.5 1.5 1.5 1.5 1.5 1.5 1.5 1.5 1.5 1.5 1.5 1.5 1.5 1.5 1.5 1.5 1.5 1.5;1.5 1.5 1.5 1.5 1.5 1.5 1.5 1.5 1.5 1.5 1.5 1.5 1.5 1.5 1.5 1.5 1.5 1.5 1.5 1.5 1.5;1.5 1.5 1.5 1.5 1.5 1.5 1.5 1.5 1.5 1.5 1.5 1.5 1.5 1.5 1.5 1.5 1.5 1.5 1.5 1.5 1.5;1.5 1.5 1.5 1.5 1.5 1.5 1.5 1.5 1.5 1.5 1.5 1.5 1.5 1.5 1.5 1.5 1.5 1.5 1.5 1.5 1.5;1.5 1.5 1.5 1.5 1.5 1.5 1.5 1.5 1.5 1.5 1.5 1.5 1.5 1.5 1.5 1.5 1.5 1.5 1.5 1.5 1.5;1.5 1.5 1.5 1.5 1.5 1.5 1.5 1.5 1.5 1.5 1.5 1.5 1.5 1.5 1.5 1.5 1.5 1.5 1.5 1.5 1.5;1.5 1.5 1.5 1.5 1.5 1.5 1.5 1.5 1.5 1.5 1.5 1.5 1.5 1.5 1.5 1.5 1.5 1.5 1.5 1.5 1.5;1.5 1.5 1.5 1.5 1.5 1.5 1.5 1.5 1.5 1.5 1.5 1.5 1.5 1.5 1.5 1.5 1.5 1.5 1.5 1.5 1.5;1.5 1.5 1.5 1.5 1.5 1.5 1.5 1.5 1.5 1.5 1.5 1.5 1.5 1.5 1.5 1.5 1.5 1.5 1.5 1.5 1.5;1.5 1.5 1.5 1.5 1.5 1.5 1.5 1.5 1.5 1.5 1.5 1.5 1.5 1.5 1.5 1.5 1.5 1.5 1.5 1.5 1.5;1.5 1.5 1.5 1.5 1.5 1.5 1.5 1.5 1.5 1.5 1.5 1.5 1.5 1.5 1.5 1.5 1.5 1.5 1.5 1.5 1.5;1.5 1.5 1.5 1.5 1.5 1.5 1.5 1.5 1.5 1.5 1.5 1.5 1.5 1.5 1.5 1.5 1.5 1.5 1.5 1.5 1.5;1.5 1.5 1.5 1.5 1.5 1.5 1.5 1.5 1.5 1.5 1.5 1.5 1.5 1.5 1.5 1.5 1.5 1.5 1.5 1.5 1.5;1.5 1.5 1.5 1.5 1.5 1.5 1.5 1.5 1.5 1.5 1.5 1.5 1.5 1.5 1.5 1.5 1.5 1.5 1.5 1.5 1.5;1.5 1.5 1.5 1.5 1.5 1.5 1.5 1.5 1.5 1.5 1.5 1.5 1.5 1.5 1.5 1.5 1.5 1.5 1.5 1.5 1.5;1.5 1.5 1.5 1.5 1.5 1.5 1.5 1.5 1.5 1.5 1.5 1.5 1.5 1.5 1.5 1.5 1.5 1.5 1.5 1.5 1.5;1.5 1.5 1.5 1.5 1.5 1.5 1.5 1.5 1.5 1.5 1.5 1.5 1.5 1.5 1.5 1.5 1.5 1.5 1.5 1.5 1.5;1.5 1.5 1.5 1.5 1.5 1.5 1.5 1.5 1.5 1.5 1.5 1.5 1.5 1.5 1.5 1.5 1.5 1.5 1.5 1.5 1.5;1.5 1.5 1.5 1.5 1.5 1.5 1.5 1.5 1.5 1.5 1.5 1.5 1.5 1.5 1.5 1.5 1.5 1.5 1.5 1.5 1.5;1.5 1.5 1.5 1.5 1.5 1.5 1.5 1.5 1.5 1.5 1.5 1.5 1.5 1.5 1.5 1.5 1.5 1.5 1.5 1.5 1.5;1.5 1.5 1.5 1.5 1.5 1.5 1.5 1.5 1.5 1.5 1.5 1.5 1.5 1.5 1.5 1.5 1.5 1.5 1.5 1.5 1.5;1.5 1.5 1.5 1.5 1.5 1.5 1.5 1.5 1.5 1.5 1.5 1.5 1.5 1.5 1.5 1.5 1.5 1.5 1.5 1.5 1.5],[1.9 1.9 1.9 1.9 1.9 1.9 1.9 1.9 1.9 1.9 1.9 1.9 1.9 1.9 1.9 1.9 1.9 1.9 1.9 1.9 1.9;1.9 1.9 1.9 1.9 1.9 1.9 1.9 1.9 1.9 1.9 1.9 1.9 1.9 1.9 1.9 1.9 1.9 1.9 1.9 1.9 1.9;1.9 1.9 1.9 1.9 1.9 1.9 1.9 1.9 1.9 1.9 1.9 1.9 1.9 1.9 1.9 1.9 1.9 1.9 1.9 1.9 1.9;1.9 1.9 1.9 1.9 1.9 1.9 1.9 1.9 1.9 1.9 1.9 1.9 1.9 1.9 1.9 1.9 1.9 1.9 1.9 1.9 1.9;1.9 1.9 1.9 1.9 1.9 1.9 1.9 1.9 1.9 1.9 1.9 1.9 1.9 1.9 1.9 1.9 1.9 1.9 1.9 1.9 1.9;1.9 1.9 1.9 1.9 1.9 1.9 1.9 1.9 1.9 1.9 1.9 1.9 1.9 1.9 1.9 1.9 1.9 1.9 1.9 1.9 1.9;1.9 1.9 1.9 1.9 1.9 1.9 1.9 1.9 1.9 1.9 1.9 1.9 1.9 1.9 1.9 1.9 1.9 1.9 1.9 1.9 1.9 ...(+1680 chars)])  CalLossMapData={'BaseCageProjectFileName','';'BaseMbcProjectFileName','';'TaskName','Calibrate Motor Loss Map';'ChildTasks',{{'DataName','';'TaskName','Import Loss Data'},{'TaskName','Generate Response Models'},{'TaskName','Generate Calibration'},{'TaskName','Update Block Parameters'}}}  CalLossWithTempMapData={}  aMode=6  RefBlkName='autolibmappedmotor/Mapped Motor'
  EMTrq : Outport  VectorParamsAs1DForOutWhenUnconnected=off
  EMCurr : Outport  Port=2  VectorParamsAs1DForOutWhenUnconnected=off
  Info : Outport  Port=3
  wires:
  BusVolt/1 -> Mapped Motor/1
  EMSpd/1 -> Mapped Motor/2
  EMTrqCmd/1 -> Mapped Motor/3
  Mapped Motor/1 -> Info/1
  Mapped Motor/2 -> EMCurr/1
  Mapped Motor/3 -> EMTrq/1
